simulink model "lab5"  (Simulink 7.3)
settings: Solver=ode45  StartTime=0.0  StopTime=10.0  RelTol=1e-3
libraries: simulink x1
settings Model: Creator=user_ftk10  LastModifiedBy=user_ftk10

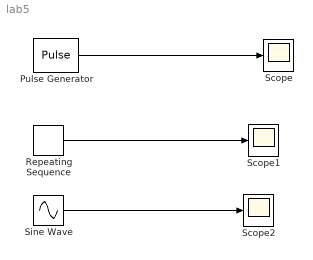
== system lab5 ==
  Pulse Generator : DiscretePulseGenerator  Amplitude=3  Period=100  PulseWidth=50  PhaseDelay=0  SampleTime=0.01
  Repeating Sequence : simulink/Sources/Repeating Sequence  SystemSampleTime=-1  rep_seq_t=[0 2]  rep_seq_y=[0 2]
  Scope : Scope
  Scope1 : Scope
  Scope2 : Scope
      settings: SaveName=ScopeData2
  Sine Wave : Sin  SineType=Sample based  Amplitude=1  Bias=0  Frequency=1  Phase=0  Samples=30  SampleTime=0.05  Offset=0
  wires:
  Repeating Sequence/1 -> Scope1/1
  Pulse Generator/1 -> Scope/1
  Sine Wave/1 -> Scope2/1
